simulink model "MultiMicrogrid"  (R2022b)
settings: Solver=ode45  StartTime=0.0  StopTime=1000  RelTol=1e-3  AbsTol=1e-5
values from neighbouring files (symbols this model uses):
  a_hidden_weights1 = zeros(n,h)    [Weights.m]
  a_hidden_weights2 = zeros(n,h)    [Weights.m]
  a_hidden_weights3 = zeros(n,h)    [Weights.m]
  a_input_weights1 = zeros(h,m)    [Weights.m]
  a_input_weights2 = zeros(h,m)    [Weights.m]
  a_input_weights3 = zeros(h,m)    [Weights.m]
  c_hidden_weights11 = zeros(100,1000)    [Training.m]
  c_hidden_weights12 = -1+(1+1)*rand(1,100,'single')    [Training.m]
  c_hidden_weights21 = zeros(100,1000)    [Training.m]
  c_hidden_weights22 = -1+(1+1)*rand(1,100,'single')    [Training.m]
  c_hidden_weights31 = zeros(100,1000)    [Training.m]
  c_hidden_weights32 = -1+(1+1)*rand(1,100,'single')    [Training.m]
  c_hidden_weights_a1 = -1+(1+1)*rand(1,100,'single')    [Training.m]
  c_hidden_weights_a2 = -1+(1+1)*rand(1,100,'single')    [Training.m]
  c_hidden_weights_a3 = -1+(1+1)*rand(1,100,'single')    [Training.m]
  c_input_weights1 = zeros(1000,m)    [Training.m]
  c_input_weights2 = zeros(1000,m)    [Training.m]
  c_input_weights3 = zeros(1000,m)    [Training.m]
  c_input_weights_a1 = zeros(100,n)    [Training.m]
  c_input_weights_a2 = zeros(100,n)    [Training.m]
  c_input_weights_a3 = zeros(100,n)    [Training.m]
libraries: simulink x27, fuzblock x3, mpclib x3, slpidlib x3
(part 2 of 2)

== system MultiMicrogrid/Agent 1 ==
  error : Inport
  Gamma : Subsystem
  generate observations : Subsystem
  Action : Outport
  wires:
  error/1 -> Gamma/2(error), generate observations/1(error)
  generate observations/1(observations) -> Gamma/1(observations)
  Gamma/1(Action) -> Action/1

== system MultiMicrogrid/Agent 2 ==
  error : Inport
  Gamma : Subsystem
  generate observations : Subsystem
  Action : Outport
  wires:
  error/1 -> Gamma/2(error), generate observations/1(error)
  generate observations/1(observations) -> Gamma/1(observations)
  Gamma/1(Action) -> Action/1

== system MultiMicrogrid/Agent 3 ==
  error : Inport
  Gamma : Subsystem
  generate observations : Subsystem
  Action : Outport
  wires:
  error/1 -> Gamma/2(error), generate observations/1(error)
  generate observations/1(observations) -> Gamma/1(observations)
  Gamma/1(Action) -> Action/1

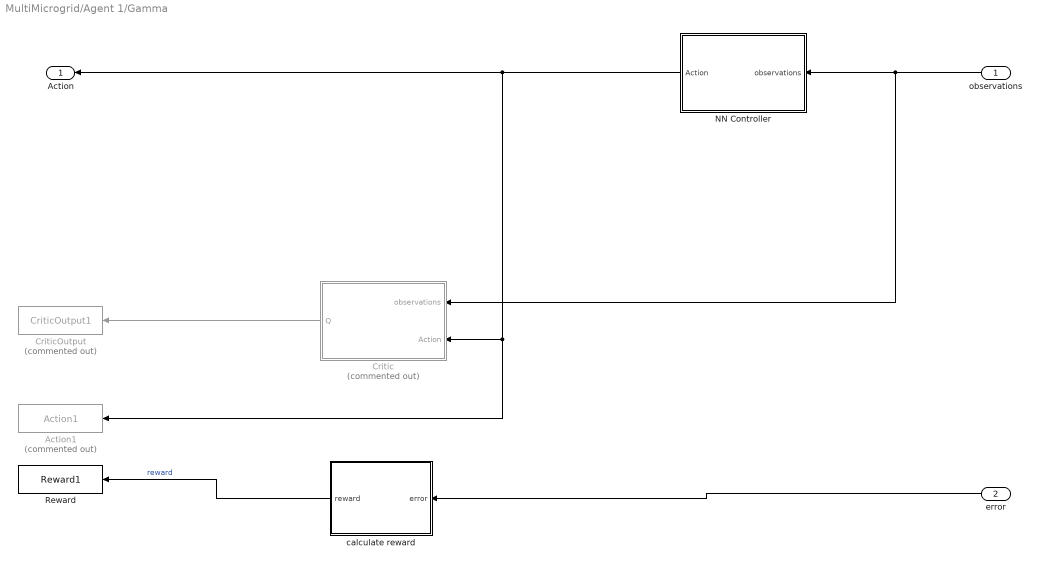
== system MultiMicrogrid/Agent 1/Gamma ==
  observations : Inport
  error : Inport  Port=2
  Action1 : ToWorkspace  Commented=on  VariableName=Action1  SampleTime=1
      settings: Save2DSignal=2-D array (concatenate along first dimension)
  Critic : Subsystem  Commented=on
  CriticOutput : ToWorkspace  Commented=on  VariableName=CriticOutput1  SampleTime=1
      settings: Save2DSignal=2-D array (concatenate along first dimension)
  NN Controller : Subsystem
  Reward : ToWorkspace  VariableName=Reward1  SampleTime=1
      settings: Save2DSignal=2-D array (concatenate along first dimension)
  calculate reward : Subsystem
  Action : Outport
  wires:
  NN Controller/1(Action) -> Action1/1, Critic/2(Action), Action/1
  observations/1 -> Critic/1(observations), NN Controller/1(observations)
  calculate reward/1(reward) -> Reward/1  "reward"
  Critic/1(Q) -> CriticOutput/1
  error/1 -> calculate reward/1(error)

== system MultiMicrogrid/Agent 1/generate observations ==
  error : Inport
  Derivative : Derivative
  Integrator : Integrator  IgnoreLimit=on
  Mux : Mux  Inputs=3
  observations : Outport  VectorParamsAs1DForOutWhenUnconnected=off
  wires:
  Mux/1 -> observations/1
  error/1 -> Derivative/1, Integrator/1, Mux/1
  Integrator/1 -> Mux/2
  Derivative/1 -> Mux/3

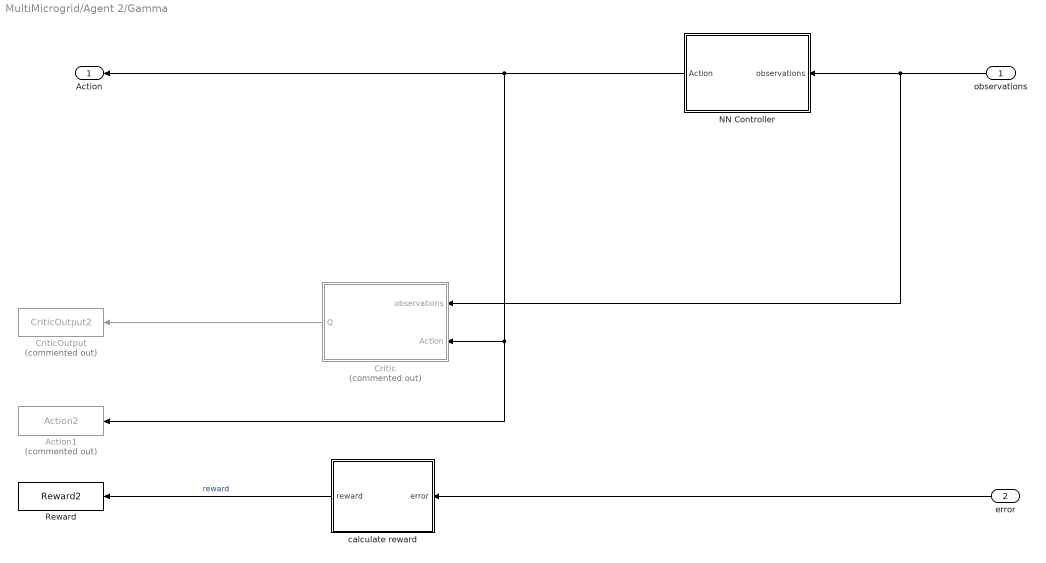
== system MultiMicrogrid/Agent 2/Gamma ==
  observations : Inport
  error : Inport  Port=2
  Action1 : ToWorkspace  Commented=on  VariableName=Action2  SampleTime=1
      settings: Save2DSignal=2-D array (concatenate along first dimension)
  Critic : Subsystem  Commented=on
  CriticOutput : ToWorkspace  Commented=on  VariableName=CriticOutput2  SampleTime=1
      settings: Save2DSignal=2-D array (concatenate along first dimension)
  NN Controller : Subsystem
  Reward : ToWorkspace  VariableName=Reward2  SampleTime=1
      settings: Save2DSignal=2-D array (concatenate along first dimension)
  calculate reward : Subsystem
  Action : Outport
  wires:
  NN Controller/1(Action) -> Action1/1, Critic/2(Action), Action/1
  observations/1 -> Critic/1(observations), NN Controller/1(observations)
  calculate reward/1(reward) -> Reward/1  "reward"
  Critic/1(Q) -> CriticOutput/1
  error/1 -> calculate reward/1(error)

== system MultiMicrogrid/Agent 2/generate observations ==
  error : Inport
  Derivative : Derivative
  Integrator : Integrator  IgnoreLimit=on
  Mux : Mux  Inputs=3
  observations : Outport  VectorParamsAs1DForOutWhenUnconnected=off
  wires:
  Mux/1 -> observations/1
  error/1 -> Derivative/1, Integrator/1, Mux/1
  Integrator/1 -> Mux/2
  Derivative/1 -> Mux/3

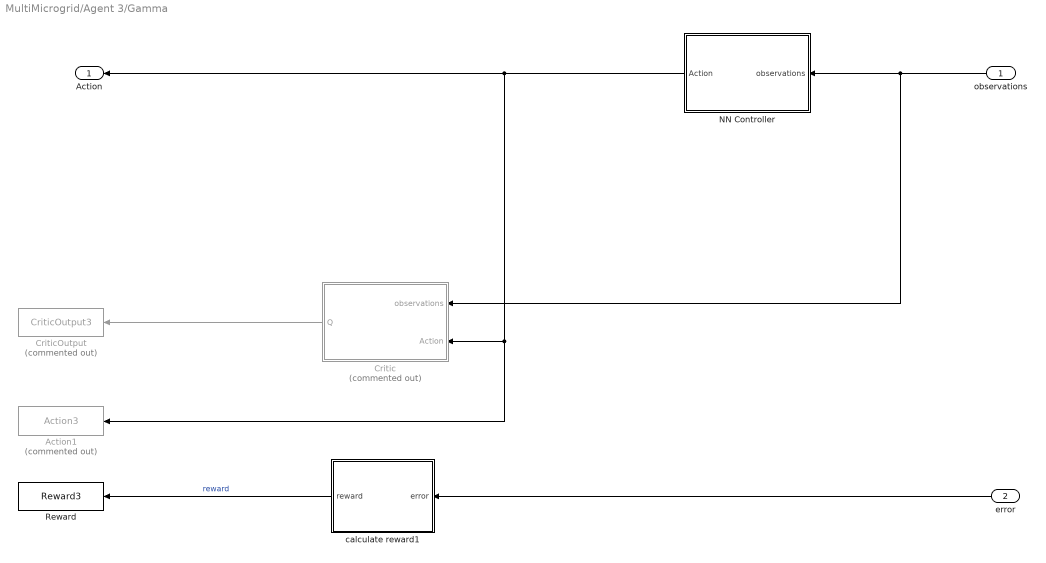
== system MultiMicrogrid/Agent 3/Gamma ==
  observations : Inport
  error : Inport  Port=2
  Action1 : ToWorkspace  Commented=on  VariableName=Action3  SampleTime=1
      settings: Save2DSignal=2-D array (concatenate along first dimension)
  Critic : Subsystem  Commented=on
  CriticOutput : ToWorkspace  Commented=on  VariableName=CriticOutput3  SampleTime=1
      settings: Save2DSignal=2-D array (concatenate along first dimension)
  NN Controller : Subsystem
  Reward : ToWorkspace  VariableName=Reward3  SampleTime=1
      settings: Save2DSignal=2-D array (concatenate along first dimension)
  calculate reward1 : Subsystem
  Action : Outport
  wires:
  NN Controller/1(Action) -> Action1/1, Critic/2(Action), Action/1
  observations/1 -> Critic/1(observations), NN Controller/1(observations)
  calculate reward1/1(reward) -> Reward/1  "reward"
  Critic/1(Q) -> CriticOutput/1
  error/1 -> calculate reward1/1(error)

== system MultiMicrogrid/Agent 3/generate observations ==
  error : Inport
  Derivative : Derivative
  Integrator : Integrator  IgnoreLimit=on
  Mux : Mux  Inputs=3
  observations : Outport  VectorParamsAs1DForOutWhenUnconnected=off
  wires:
  Mux/1 -> observations/1
  error/1 -> Derivative/1, Integrator/1, Mux/1
  Integrator/1 -> Mux/2
  Derivative/1 -> Mux/3

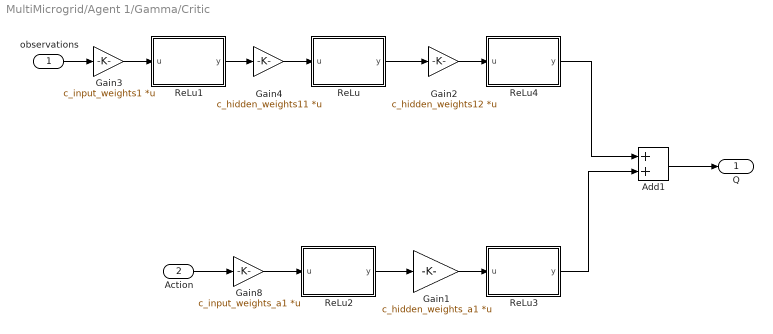
== system MultiMicrogrid/Agent 1/Gamma/Critic ==
  observations : Inport
  Action : Inport  Port=2
  Add1 : Sum
  Gain1 : Gain  Gain=c_hidden_weights_a1  Multiplication=Matrix(K*u)
  Gain2 : Gain  Gain=c_hidden_weights12  Multiplication=Matrix(K*u)
  Gain3 : Gain  Gain=c_input_weights1  Multiplication=Matrix(K*u)
  Gain4 : Gain  Gain=c_hidden_weights11  Multiplication=Matrix(K*u)
  Gain8 : Gain  Gain=c_input_weights_a1  Multiplication=Matrix(K*u)
  ReLu : MATLAB Function  TreatAsAtomicUnit=on
  ReLu1 : MATLAB Function  TreatAsAtomicUnit=on
  ReLu2 : MATLAB Function  TreatAsAtomicUnit=on
  ReLu3 : MATLAB Function  TreatAsAtomicUnit=on
  ReLu4 : MATLAB Function  TreatAsAtomicUnit=on
  Q : Outport
  wires:
  observations/1 -> Gain3/1
  Add1/1 -> Q/1
  Action/1 -> Gain8/1
  ReLu3/1(y) -> Add1/2
  Gain8/1 -> ReLu2/1(u)
  ReLu2/1(y) -> Gain1/1
  Gain1/1 -> ReLu3/1(u)
  Gain3/1 -> ReLu1/1(u)
  ReLu1/1(y) -> Gain4/1
  Gain4/1 -> ReLu/1(u)
  ReLu/1(y) -> Gain2/1
  Gain2/1 -> ReLu4/1(u)
  ReLu4/1(y) -> Add1/1

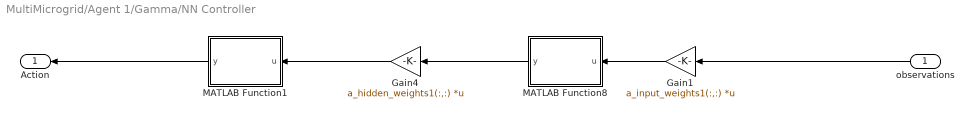
== system MultiMicrogrid/Agent 1/Gamma/NN Controller ==
  observations : Inport
  Gain1 : Gain  Gain=a_input_weights1(:,:)  Multiplication=Matrix(K*u)
  Gain4 : Gain  Gain=a_hidden_weights1(:,:)  Multiplication=Matrix(K*u)
  MATLAB Function1 : MATLAB Function  TreatAsAtomicUnit=on
  MATLAB Function8 : MATLAB Function  TreatAsAtomicUnit=on
  Action : Outport
  wires:
  Gain1/1 -> MATLAB Function8/1(u)
  Gain4/1 -> MATLAB Function1/1(u)
  MATLAB Function8/1(y) -> Gain4/1
  observations/1 -> Gain1/1
  MATLAB Function1/1(y) -> Action/1

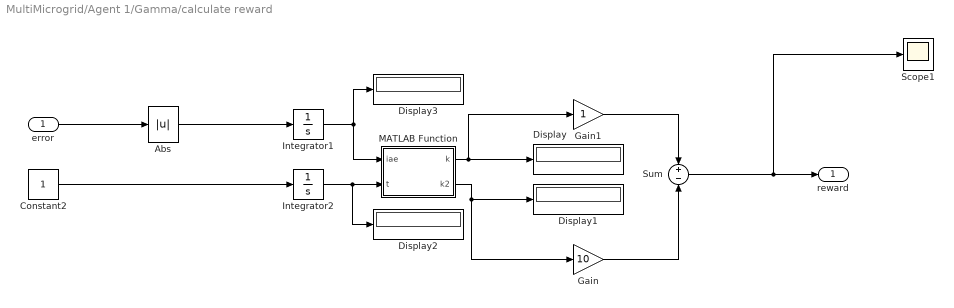
== system MultiMicrogrid/Agent 1/Gamma/calculate reward ==
  error : Inport
  Abs : Abs  SaturateOnIntegerOverflow=off
  Constant2 : Constant  SampleTime=1
  Display{,1..3} (4 alike) : Display
  Gain : Gain  Gain=10
  Gain1 : Gain
  Integrator1 : Integrator
  Integrator2 : Integrator
  MATLAB Function : MATLAB Function  TreatAsAtomicUnit=on
  Scope1 : Scope
  Sum : Sum  Inputs=+-
  reward : Outport  VectorParamsAs1DForOutWhenUnconnected=off
  wires:
  error/1 -> Abs/1
  Abs/1 -> Integrator1/1
  Integrator1/1 -> Display3/1, MATLAB Function/1(iae)
  Integrator2/1 -> Display2/1, MATLAB Function/2(t)
  Constant2/1 -> Integrator2/1
  MATLAB Function/1(k) -> Display/1, Gain1/1
  MATLAB Function/2(k2) -> Gain/1, Display1/1
  Gain/1 -> Sum/2
  Gain1/1 -> Sum/1
  Sum/1 -> Scope1/1, reward/1

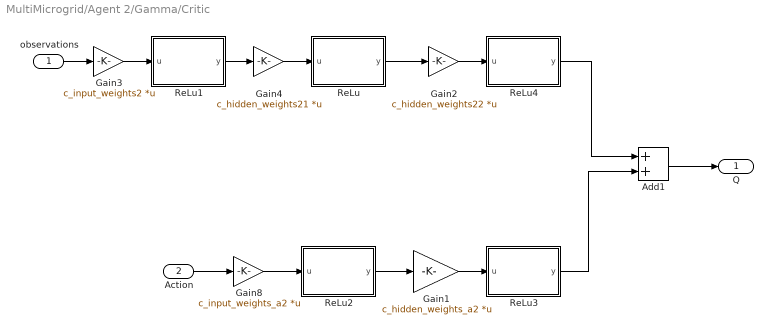
== system MultiMicrogrid/Agent 2/Gamma/Critic ==
  observations : Inport
  Action : Inport  Port=2
  Add1 : Sum
  Gain1 : Gain  Gain=c_hidden_weights_a2  Multiplication=Matrix(K*u)
  Gain2 : Gain  Gain=c_hidden_weights22  Multiplication=Matrix(K*u)
  Gain3 : Gain  Gain=c_input_weights2  Multiplication=Matrix(K*u)
  Gain4 : Gain  Gain=c_hidden_weights21  Multiplication=Matrix(K*u)
  Gain8 : Gain  Gain=c_input_weights_a2  Multiplication=Matrix(K*u)
  ReLu : MATLAB Function  TreatAsAtomicUnit=on
  ReLu1 : MATLAB Function  TreatAsAtomicUnit=on
  ReLu2 : MATLAB Function  TreatAsAtomicUnit=on
  ReLu3 : MATLAB Function  TreatAsAtomicUnit=on
  ReLu4 : MATLAB Function  TreatAsAtomicUnit=on
  Q : Outport
  wires:
  observations/1 -> Gain3/1
  Add1/1 -> Q/1
  Action/1 -> Gain8/1
  ReLu3/1(y) -> Add1/2
  Gain8/1 -> ReLu2/1(u)
  ReLu2/1(y) -> Gain1/1
  Gain1/1 -> ReLu3/1(u)
  Gain3/1 -> ReLu1/1(u)
  ReLu1/1(y) -> Gain4/1
  Gain4/1 -> ReLu/1(u)
  ReLu/1(y) -> Gain2/1
  Gain2/1 -> ReLu4/1(u)
  ReLu4/1(y) -> Add1/1

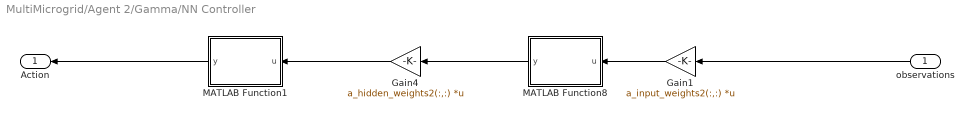
== system MultiMicrogrid/Agent 2/Gamma/NN Controller ==
  observations : Inport
  Gain1 : Gain  Gain=a_input_weights2(:,:)  Multiplication=Matrix(K*u)
  Gain4 : Gain  Gain=a_hidden_weights2(:,:)  Multiplication=Matrix(K*u)
  MATLAB Function1 : MATLAB Function  TreatAsAtomicUnit=on
  MATLAB Function8 : MATLAB Function  TreatAsAtomicUnit=on
  Action : Outport
  wires:
  Gain1/1 -> MATLAB Function8/1(u)
  Gain4/1 -> MATLAB Function1/1(u)
  MATLAB Function8/1(y) -> Gain4/1
  observations/1 -> Gain1/1
  MATLAB Function1/1(y) -> Action/1

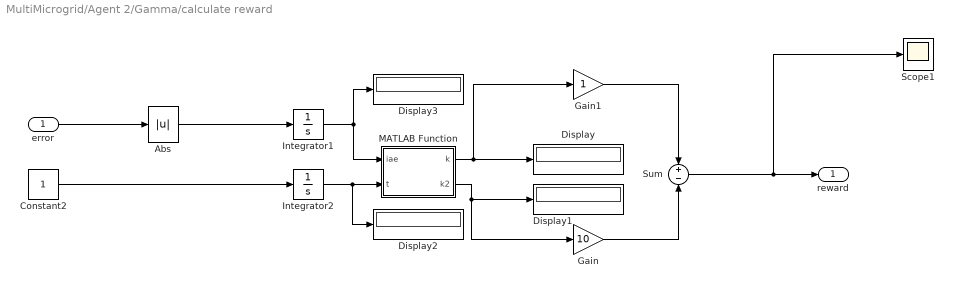
== system MultiMicrogrid/Agent 2/Gamma/calculate reward ==
  error : Inport
  Abs : Abs  SaturateOnIntegerOverflow=off
  Constant2 : Constant
  Display{,1..3} (4 alike) : Display
  Gain : Gain  Gain=10
  Gain1 : Gain
  Integrator1 : Integrator
  Integrator2 : Integrator
  MATLAB Function : MATLAB Function  TreatAsAtomicUnit=on
  Scope1 : Scope
  Sum : Sum  Inputs=+-
  reward : Outport  VectorParamsAs1DForOutWhenUnconnected=off
  wires:
  error/1 -> Abs/1
  Abs/1 -> Integrator1/1
  Integrator1/1 -> Display3/1, MATLAB Function/1(iae)
  Integrator2/1 -> Display2/1, MATLAB Function/2(t)
  Constant2/1 -> Integrator2/1
  MATLAB Function/1(k) -> Display/1, Gain1/1
  MATLAB Function/2(k2) -> Gain/1, Display1/1
  Sum/1 -> Scope1/1, reward/1
  Gain/1 -> Sum/2
  Gain1/1 -> Sum/1

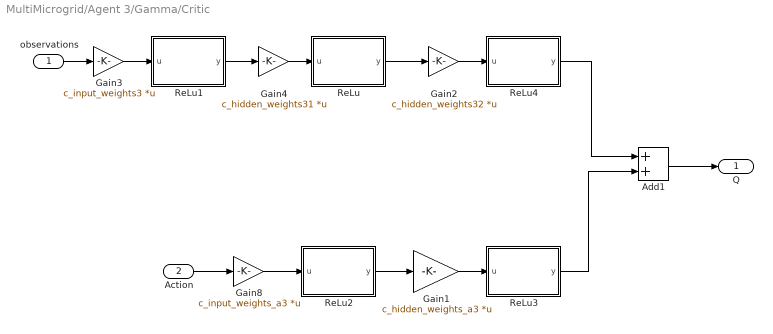
== system MultiMicrogrid/Agent 3/Gamma/Critic ==
  observations : Inport
  Action : Inport  Port=2
  Add1 : Sum
  Gain1 : Gain  Gain=c_hidden_weights_a3  Multiplication=Matrix(K*u)
  Gain2 : Gain  Gain=c_hidden_weights32  Multiplication=Matrix(K*u)
  Gain3 : Gain  Gain=c_input_weights3  Multiplication=Matrix(K*u)
  Gain4 : Gain  Gain=c_hidden_weights31  Multiplication=Matrix(K*u)
  Gain8 : Gain  Gain=c_input_weights_a3  Multiplication=Matrix(K*u)
  ReLu : MATLAB Function  TreatAsAtomicUnit=on
  ReLu1 : MATLAB Function  TreatAsAtomicUnit=on
  ReLu2 : MATLAB Function  TreatAsAtomicUnit=on
  ReLu3 : MATLAB Function  TreatAsAtomicUnit=on
  ReLu4 : MATLAB Function  TreatAsAtomicUnit=on
  Q : Outport
  wires:
  observations/1 -> Gain3/1
  Add1/1 -> Q/1
  Action/1 -> Gain8/1
  ReLu3/1(y) -> Add1/2
  Gain8/1 -> ReLu2/1(u)
  ReLu2/1(y) -> Gain1/1
  Gain1/1 -> ReLu3/1(u)
  Gain3/1 -> ReLu1/1(u)
  ReLu1/1(y) -> Gain4/1
  Gain4/1 -> ReLu/1(u)
  ReLu/1(y) -> Gain2/1
  Gain2/1 -> ReLu4/1(u)
  ReLu4/1(y) -> Add1/1

== system MultiMicrogrid/Agent 3/Gamma/NN Controller ==
  observations : Inport
  Gain1 : Gain  Gain=a_input_weights3(:,:)  Multiplication=Matrix(K*u)
  Gain4 : Gain  Gain=a_hidden_weights3(:,:)  Multiplication=Matrix(K*u)
  MATLAB Function1 : MATLAB Function  TreatAsAtomicUnit=on
  MATLAB Function8 : MATLAB Function  TreatAsAtomicUnit=on
  Action : Outport
  wires:
  Gain1/1 -> MATLAB Function8/1(u)
  Gain4/1 -> MATLAB Function1/1(u)
  MATLAB Function8/1(y) -> Gain4/1
  observations/1 -> Gain1/1
  MATLAB Function1/1(y) -> Action/1

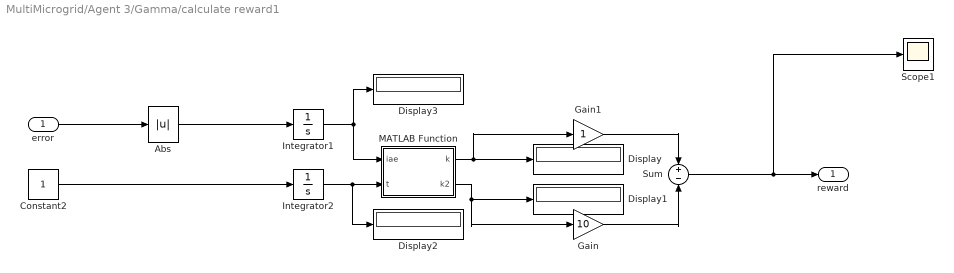
== system MultiMicrogrid/Agent 3/Gamma/calculate reward1 ==
  error : Inport
  Abs : Abs  SaturateOnIntegerOverflow=off
  Constant2 : Constant
  Display{,1..3} (4 alike) : Display
  Gain : Gain  Gain=10
  Gain1 : Gain
  Integrator1 : Integrator
  Integrator2 : Integrator
  MATLAB Function : MATLAB Function  TreatAsAtomicUnit=on
  Scope1 : Scope
  Sum : Sum  Inputs=+-
  reward : Outport  VectorParamsAs1DForOutWhenUnconnected=off
  wires:
  error/1 -> Abs/1
  Abs/1 -> Integrator1/1
  Integrator1/1 -> Display3/1, MATLAB Function/1(iae)
  Integrator2/1 -> Display2/1, MATLAB Function/2(t)
  Constant2/1 -> Integrator2/1
  MATLAB Function/1(k) -> Display/1, Gain1/1
  MATLAB Function/2(k2) -> Gain/1, Display1/1
  Sum/1 -> Scope1/1, reward/1
  Gain/1 -> Sum/2
  Gain1/1 -> Sum/1

== matlab function MultiMicrogrid/Agent 1/Gamma/NN Controller/MATLAB Function8 ==
  data: u input; y output
function y = fcn(u)
y=ones(size(u));
for i=1:3
y(i)=(4/(1+exp(-3*u(i)))-2);
end
end

== matlab function MultiMicrogrid/Agent 2/Gamma/NN Controller/MATLAB Function1 ==
  data: u input; y output
function y = fcn(u)
y=ones(size(u));
for i=1:1
y(i)=(8/(1+exp(-4*u(i)))-4);
end
end

== matlab function MultiMicrogrid/Agent 2/Gamma/NN Controller/MATLAB Function8 ==
  data: u input; y output
function y = fcn(u)
y=ones(size(u));
for i=1:3
y(i)=(8/(1+exp(-4*u(i)))-4);
end
end

== matlab function MultiMicrogrid/Agent 2/Gamma/Critic/ReLu ==
  data: u input; y output
function y = fcn(u)
y=ones(size(u));
for i=1:100
 if u>0
    y(i)=u(i);
 else
    y(i)=u(i)*0.01;
 end
end

end

== matlab function MultiMicrogrid/Agent 2/Gamma/Critic/ReLu1 ==
  data: u input; y output
function y = fcn(u)
y=ones(size(u));
for i=1:1000
 if u>0
    y(i)=u(i);
 else
    y(i)=u(i)*0.01;
 end
end

end

== matlab function MultiMicrogrid/Agent 2/Gamma/calculate reward/MATLAB Function ==
  data: iae input; k output; t input; k2 output
function [k,k2] = fcn(iae,t)
k = (t)/((iae^2+t^2)^(1/2));
k2 = (iae)/((iae^2+t^2)^(1/2));
end

== matlab function MultiMicrogrid/Agent 3/Gamma/calculate reward1/MATLAB Function ==
  data: iae input; k output; t input; k2 output
function [k,k2] = fcn(iae,t)
k = (t)/((iae^2+t^2)^(1/2));
k2 = (iae)/((iae^2+t^2)^(1/2));
end

== matlab function MultiMicrogrid/Agent 1/Gamma/calculate reward/MATLAB Function ==
  data: iae input; k output; t input; k2 output
function [k,k2] = fcn(iae,t)
k = (t)/((iae^2+t^2)^(1/2));
k2 = (iae)/((iae^2+t^2)^(1/2));
end

== matlab function MultiMicrogrid/Agent 3/Gamma/Critic/ReLu1 ==
  data: u input; y output
function y = fcn(u)
y=ones(size(u));
for i=1:1000
 if u>0
    y(i)=u(i);
 else
    y(i)=u(i)*0.01;
 end
end

end

== matlab function MultiMicrogrid/Agent 2/Gamma/Critic/ReLu2 ==
  data: u input; y output
function y = fcn(u)
y=ones(size(u));
for i=1:100
 if u>0
    y(i)=u(i);
 else
    y(i)=u(i)*0.01;
 end
end

end

== matlab function MultiMicrogrid/Agent 2/Gamma/Critic/ReLu3 ==
  data: u input; y output
function y = fcn(u)
y=ones(size(u));
for i=1:1
 if u>0
    y(i)=u(i);
 else
    y(i)=u(i)*0.01;
 end
end

end

== matlab function MultiMicrogrid/Agent 2/Gamma/Critic/ReLu4 ==
  data: u input; y output
function y = fcn(u)
y=ones(size(u));
for i=1:1
 if u>0
    y(i)=u(i);
 else
    y(i)=u(i)*0.01;
 end
end

end

== matlab function MultiMicrogrid/Agent 3/Gamma/Critic/ReLu2 ==
  data: u input; y output
function y = fcn(u)
y=ones(size(u));
for i=1:100
 if u>0
    y(i)=u(i);
 else
    y(i)=u(i)*0.01;
 end
end

end

== matlab function MultiMicrogrid/Agent 3/Gamma/Critic/ReLu3 ==
  data: u input; y output
function y = fcn(u)
y=ones(size(u));
for i=1:1
 if u>0
    y(i)=u(i);
 else
    y(i)=u(i)*0.01;
 end
end

end

== matlab function MultiMicrogrid/Agent 3/Gamma/Critic/ReLu4 ==
  data: u input; y output
function y = fcn(u)
y=ones(size(u));
for i=1:1
 if u>0
    y(i)=u(i);
 else
    y(i)=u(i)*0.01;
 end
end

end

== matlab function MultiMicrogrid/Agent 3/Gamma/NN Controller/MATLAB Function1 ==
  data: u input; y output
function y = fcn(u)
y=ones(size(u));
for i=1:1
y(i)=(4/(1+exp(-3*u(i)))-2);
end
end

== matlab function MultiMicrogrid/Agent 3/Gamma/NN Controller/MATLAB Function8 ==
  data: u input; y output
function y = fcn(u)
y=ones(size(u));
for i=1:3
y(i)=(4/(1+exp(-3*u(i)))-2);
end
end

== matlab function MultiMicrogrid/Agent 1/Gamma/Critic/ReLu ==
  data: u input; y output
function y = fcn(u)
y=ones(size(u));
for i=1:100
 if u>0
    y(i)=u(i);
 else
    y(i)=u(i)*0.01;
 end
end

end

== matlab function MultiMicrogrid/Agent 1/Gamma/Critic/ReLu1 ==
  data: u input; y output
function y = fcn(u)
y=ones(size(u));
for i=1:1000
 if u>0
    y(i)=u(i);
 else
    y(i)=u(i)*0.01;
 end
end

end

== matlab function MultiMicrogrid/Agent 1/Gamma/Critic/ReLu2 ==
  data: u input; y output
function y = fcn(u)
y=ones(size(u));
for i=1:100
 if u>0
    y(i)=u(i);
 else
    y(i)=u(i)*0.01;
 end
end

end

== matlab function MultiMicrogrid/Agent 1/Gamma/Critic/ReLu3 ==
  data: u input; y output
function y = fcn(u)
y=ones(size(u));
for i=1:1
 if u>0
    y(i)=u(i);
 else
    y(i)=u(i)*0.01;
 end
end

end

== matlab function MultiMicrogrid/Agent 1/Gamma/Critic/ReLu4 ==
  data: u input; y output
function y = fcn(u)
y=ones(size(u));
for i=1:1
 if u>0
    y(i)=u(i);
 else
    y(i)=u(i)*0.01;
 end
end

end

== matlab function MultiMicrogrid/Agent 3/Gamma/Critic/ReLu ==
  data: u input; y output
function y = fcn(u)
y=ones(size(u));
for i=1:100
 if u>0
    y(i)=u(i);
 else
    y(i)=u(i)*0.01;
 end
end

end

== matlab function MultiMicrogrid/Agent 1/Gamma/NN Controller/MATLAB Function1 ==
  data: u input; y output
function y = fcn(u)
y=ones(size(u));
for i=1:1
y(i)=(4/(1+exp(-3*u(i)))-2);
end
end
